simulink model "sampleModel1695_4"  (R2023a)
settings: Solver=VariableStepAuto  StartTime=0.0  StopTime=10.0  RelTol=1e-3
libraries: simulink x3, hdlsllib x3
settings Model: Creator=user1  LastModifiedBy=user1

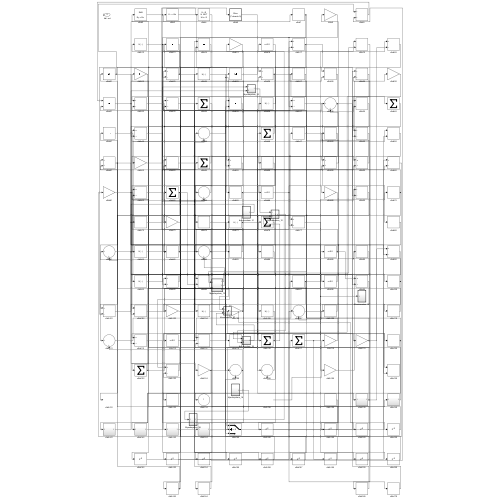
[thumbnail: Simulink's stored preview of the top-level diagram]
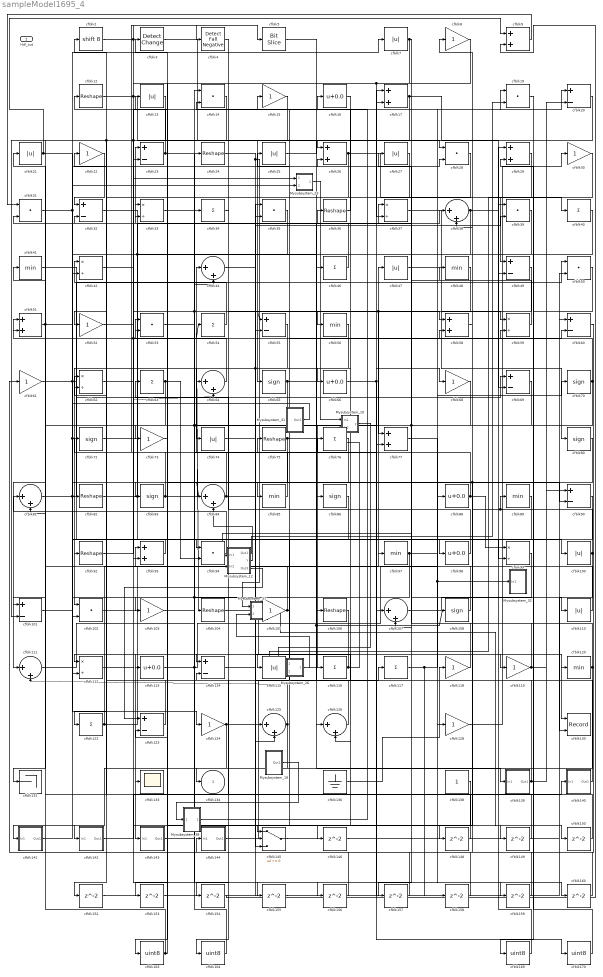
== system sampleModel1695_4 ==
  Mysubsystem_10 : Subsystem  TreatAsAtomicUnit=on  RTWFcnName=Mysubsystem_10
      settings: RTWFcnNameOpts=User specified  RTWFileNameOpts=Use function name
  Mysubsystem_12 : Subsystem  TreatAsAtomicUnit=on  RTWFcnName=Mysubsystem_12
      settings: RTWFcnNameOpts=User specified  RTWFileNameOpts=Use function name
  Mysubsystem_18 : Subsystem  TreatAsAtomicUnit=on  RTWFcnName=Mysubsystem_18
      settings: RTWFcnNameOpts=User specified  RTWFileNameOpts=Use function name
  Mysubsystem_23 : Subsystem  TreatAsAtomicUnit=on  RTWFcnName=Mysubsystem_23
      settings: RTWFcnNameOpts=User specified  RTWFileNameOpts=Use function name
  Mysubsystem_26 : Subsystem  TreatAsAtomicUnit=on  RTWFcnName=Mysubsystem_26
      settings: RTWFcnNameOpts=User specified  RTWFileNameOpts=Use function name
  Mysubsystem_31 : Subsystem  TreatAsAtomicUnit=on  RTWFcnName=Mysubsystem_31
      settings: RTWFcnNameOpts=User specified  RTWFileNameOpts=Use function name
  Mysubsystem_32 : Subsystem  TreatAsAtomicUnit=on  RTWFcnName=Mysubsystem_32
      settings: RTWFcnNameOpts=User specified  RTWFileNameOpts=Use function name
  Mysubsystem_37 : Subsystem  TreatAsAtomicUnit=on  RTWFcnName=Mysubsystem_37
      settings: RTWFcnNameOpts=User specified  RTWFileNameOpts=Use function name
  Mysubsystem_38 : Subsystem  TreatAsAtomicUnit=on  RTWFcnName=Mysubsystem_38
      settings: RTWFcnNameOpts=User specified  RTWFileNameOpts=Use function name
  cfblk{7,13,21,25,27,47,74,100,110,115} (10 alike) : Abs  OutDataTypeStr=uint8  SaturateOnIntegerOverflow=off
  cfblk{20,23,32,49,55,60,69,90,101,114,123} (11 alike) : Sum  Inputs=+-  OutDataTypeStr=uint8
  cfblk{14,19,28,31,35,39,50,53,94,102} (10 alike) : DotProduct  OutDataTypeStr=uint8
  cfblk{8,15,22,30,52,61,68,73,103,105,118..119,124,128} (14 alike) : Gain  OutDataTypeStr=uint8
  cfblk{12,24,36,75,82,92,104,106} (8 alike) : Reshape
  cfblk{38,44,64,81,84,107,111,125..126} (9 alike) : Sum  Inputs=|++  OutDataTypeStr=uint8
  cfblk{65,70,72,80,83,86,108} (7 alike) : Signum
  cfblk{33,37,42,59,62,99,112} (7 alike) : Product  Inputs=*/  OutDataTypeStr=uint8  RndMeth=Zero  SaturateOnIntegerOverflow=on
  cfblk{16,66,88,98,113} (5 alike) : Bias  Bias=0.0  SaturateOnIntegerOverflow=off
  cfblk{34,40,46,54,63,76,116..117,122} (9 alike) : Sum  Inputs=+  OutDataTypeStr=uint8
  cfblk{41,48,56,85,89,97,120} (7 alike) : MinMax  OutDataTypeStr=uint8
  cfblk130 : Record  FileSettingsInternal="{\"entries\":[{\"content\":{\"excelSettings\":{\"content\":{},\"type\":\"Streamout.ExcelSettings\"}},\"type\":\"Streamout.FileSettingStorage\",\"uuid\":\"\"}],\"packageUris\":[\"http:\\/\\/schema.mathworks.com\\/mf0\\/streamout_blocks\\/R2020a\"],\"version\":\"1.0\"}"  Layout=[1 1]  SignalsInternal="{\"entries\":[{\"content\":{\"signals\":[{\"content\":{\"blockPath\":[],\"dimensions\":[1],\"domain\":\"\",\"lineColor\":\"#a2142f\",\"plots\":[1],\"port\":1,\"signalID\":35599,\"signalName\":\"cfblk104\"},\"type\":\"RecordBlkView.Signal\",\"uuid\":\"\"},{\"content\":{\"blockPath\":[],\"dimensions\":[1],\"domain\":\"\",\"lineColor\":\"#139fff\",\"plots\":[1],\"port\":2,\"signalID\":35602,\"signalName\":\"cfblk100\"},\"type\":\"RecordBlkView.Signal\",\"uuid\":\"\"}]},\"type\":\"RecordBlkView.InputSignals\",\"uuid\":\"\"}],\"packageUris\":[\"http:\\/\\/schema.mathworks.com\\/mf0\\/streamout_blocks\\/R2020a\"],\"version\":\"1.0\"}"  VisualizationBindings="{\"xyplotplugin\":{\"info\":[{\"series\":[{\"bindingParametersList\":[{\"parameter\":\"X-Axis\",\"signalID\":35599,\"signalName\":\"cfblk104\"},{\"parameter\":\"Y-Axis\",\"signalID\":35602,\"signalName\":\"cfblk100\"}],\"seriesID\":21196}],\"subplotID\":1}]}}"  CompatibilityTag=XY  st=-1
  cfblk131 : Terminator
  cfblk133 : Scope
  cfblk136 : Ground
  cfblk138 : Constant  OutDataTypeStr=uint8  SampleTime=-1
  cfblk139 : Subsystem
      settings: LibrarySourceBlock=|
      | hdlsllib/Ports &
      | Subsystems/Subsystem
  cfblk140 : Subsystem
      settings: LibrarySourceBlock=|
      | hdlsllib/Ports &
      | Subsystems/Subsystem
  cfblk141 : Subsystem
      settings: LibrarySourceBlock=|
      | hdlsllib/Ports &
      | Subsystems/Subsystem
  cfblk142 : Subsystem
      settings: LibrarySourceBlock=|
      | hdlsllib/Ports &
      | Subsystems/Subsystem
  cfblk143 : Subsystem
      settings: LibrarySourceBlock=|
      | hdlsllib/Ports &
      | Subsystems/Subsystem
  cfblk144 : Subsystem
      settings: LibrarySourceBlock=|
      | hdlsllib/Ports &
      | Subsystems/Subsystem
  cfblk145 : Switch  OutDataTypeStr=uint8  SaturateOnIntegerOverflow=off  InputSameDT=off
  cfblk{146,148..150,152..160} (13 alike) : Delay  SampleTime=1
  cfblk{163..164,169..170} (4 alike) : DataTypeConversion  OutDataTypeStr=uint8  SaturateOnIntegerOverflow=off  RndMeth=Floor
  cfblk{9,17,26,29,51,58,77,93} (8 alike) : Sum  OutDataTypeStr=uint8
  cfblk2 : ArithShift  BitShiftNumber=8
  cfblk3 : simulink/Logic and Bit Operations/Detect Change  vinit=0  OutDataTypeStr=uint8
      settings: LibrarySourceBlock=|
      | hdlsllib/Logic and Bit
      | Operations/Detect
      | Change
  cfblk4 : hdlsllib/Logic and Bit Operations/Detect Fall Negative  vinit=0  OutDataTypeStr=uint8
  cfblk5 : hdlsllib/Logic and Bit Operations/Bit Slice  lidx=7  ridx=0
  cfblk134 : Outport  OutDataTypeStr=uint8  VectorParamsAs1DForOutWhenUnconnected=off
  Hdl_out : Outport  Port=2  OutDataTypeStr=uint8
  wires:
  cfblk119/1 -> cfblk93/1, cfblk20/2
  cfblk126/1 -> cfblk3/1
  cfblk83/1 -> cfblk5/1, cfblk17/2
  cfblk50/1 -> cfblk115/1
  cfblk85/1 -> cfblk44/1
  cfblk125/1 -> cfblk141/1(In1), cfblk111/2
  cfblk106/1 -> cfblk143/1(In1)
  cfblk102/1 -> cfblk47/1
  cfblk3/1 -> cfblk26/1
  cfblk107/1 -> cfblk110/1
  cfblk41/1 -> cfblk98/1
  cfblk81/1 -> cfblk50/1, cfblk99/2
  cfblk54/1 -> cfblk42/1
  cfblk46/1 -> cfblk23/1
  cfblk124/1 -> cfblk134/1, cfblk117/1
  cfblk139/1(Out1) -> cfblk75/1, cfblk90/1
  cfblk88/1 -> cfblk2/1, cfblk99/1
  cfblk53/1 -> cfblk34/1
  cfblk48/1 -> cfblk77/1, cfblk126/2
  cfblk145/1 -> cfblk50/2
  cfblk39/1 -> cfblk42/2
  cfblk56/1 -> cfblk102/1
  cfblk128/1 -> cfblk30/1
  cfblk138/1 -> cfblk61/1
  cfblk140/1(Out1) -> cfblk62/1
  cfblk51/1 -> cfblk111/1, cfblk83/1
  cfblk89/1 -> cfblk102/2
  cfblk8/1 -> cfblk93/2
  cfblk62/1 -> Mysubsystem_23/1(In1), cfblk54/1
  cfblk68/1 -> cfblk116/1
  cfblk117/1 -> Mysubsystem_32/1(In1), cfblk70/1, cfblk158/1
  cfblk55/1 -> cfblk104/1, cfblk145/2
  cfblk16/1 -> cfblk66/1
  cfblk58/1 -> cfblk8/1
  cfblk26/1 -> cfblk40/1, cfblk73/1
  cfblk60/1 -> cfblk144/1(In1)
  cfblk72/1 -> cfblk36/1
  cfblk30/1 -> cfblk49/1
  cfblk123/1 -> cfblk22/1
  cfblk21/1 -> cfblk9/1, cfblk124/1
  cfblk70/1 -> cfblk74/1, cfblk81/2, cfblk25/1
  cfblk37/1 -> cfblk59/1
  cfblk76/1 -> cfblk86/1
  cfblk144/1(Out1) -> cfblk46/1
  cfblk136/1 -> cfblk118/1
  cfblk86/1 -> cfblk145/1
  cfblk28/1 -> cfblk56/1
  cfblk32/1 -> cfblk106/1, cfblk126/1
  cfblk7/1 -> cfblk133/1, cfblk37/2, cfblk107/2
  cfblk23/1 -> cfblk12/1, cfblk156/1
  cfblk103/1 -> cfblk76/1
  cfblk122/1 -> Mysubsystem_12/2(In2), cfblk97/1
  cfblk110/1 -> cfblk53/1
  cfblk116/1 -> Mysubsystem_10/2(In2), cfblk112/1
  cfblk64/1 -> cfblk51/1
  cfblk66/1 -> cfblk68/1, cfblk170/1
  cfblk104/1 -> cfblk130/1
  cfblk63/1 -> cfblk82/1, cfblk94/2
  cfblk15/1 -> cfblk131/1, cfblk23/2
  cfblk120/1 -> cfblk142/1(In1), cfblk31/2
  cfblk52/1 -> cfblk26/2
  cfblk97/1 -> cfblk19/1, cfblk112/2
  cfblk12/1 -> cfblk65/1, cfblk155/1
  cfblk82/1 -> cfblk24/1, cfblk145/3
  cfblk142/1(Out1) -> cfblk140/1(In1)
  cfblk93/1 -> cfblk92/1
  cfblk25/1 -> cfblk28/1
  cfblk9/1 -> cfblk31/1
  cfblk80/1 -> cfblk84/1, cfblk148/1
  cfblk69/1 -> Mysubsystem_12/1(In1), cfblk94/1
  cfblk22/1 -> cfblk32/1
  cfblk27/1 -> cfblk52/1
  cfblk47/1 -> cfblk80/1
  cfblk40/1 -> cfblk122/1
  cfblk98/1 -> cfblk63/1
  cfblk65/1 -> cfblk101/1, cfblk139/1(In1)
  cfblk17/1 -> cfblk69/2, cfblk103/1
  cfblk94/1 -> cfblk21/1
  cfblk105/1 -> cfblk15/1, cfblk81/1
  cfblk92/1 -> cfblk20/1
  cfblk14/1 -> cfblk163/1
  cfblk59/1 -> cfblk27/1
  cfblk75/1 -> cfblk59/2, cfblk153/1
  cfblk100/1 -> cfblk89/1, cfblk48/1, cfblk130/2
  cfblk73/1 -> cfblk13/1
  cfblk5/1 -> cfblk119/1
  cfblk111/1 -> cfblk44/2
  cfblk113/1 -> cfblk88/1, cfblk58/2
  cfblk115/1 -> cfblk108/1, cfblk37/1
  cfblk2/1 -> cfblk4/1, cfblk64/2
  cfblk44/1 -> cfblk39/2
  cfblk24/1 -> Mysubsystem_37/1(In1), cfblk125/1
  cfblk74/1 -> cfblk120/1
  cfblk38/1 -> cfblk49/2, cfblk55/2
  cfblk143/1(Out1) -> cfblk38/1
  cfblk118/1 -> cfblk33/1
  cfblk13/1 -> cfblk101/2, cfblk152/1
  cfblk61/1 -> cfblk128/1, cfblk100/1
  cfblk49/1 -> cfblk114/1
  cfblk31/1 -> cfblk28/2, cfblk90/2
  cfblk33/1 -> cfblk105/1, cfblk159/1, cfblk77/2, cfblk55/1
  cfblk108/1 -> cfblk62/2
  cfblk34/1 -> cfblk64/1
  cfblk42/1 -> cfblk58/1
  cfblk36/1 -> cfblk16/1
  cfblk141/1(Out1) -> cfblk7/1
  cfblk84/1 -> cfblk72/1, cfblk60/2
  cfblk114/1 -> cfblk35/2
  cfblk35/1 -> cfblk113/1
  cfblk20/1 -> cfblk146/1
  cfblk146/1 -> cfblk39/1
  cfblk148/1 -> cfblk51/2
  cfblk149/1 -> cfblk114/2
  cfblk112/1 -> cfblk150/1
  cfblk150/1 -> cfblk32/2
  cfblk152/1 -> cfblk107/1
  cfblk153/1 -> cfblk125/2
  cfblk90/1 -> cfblk154/1
  cfblk154/1 -> cfblk9/2
  cfblk155/1 -> cfblk60/1
  cfblk156/1 -> cfblk123/2
  cfblk99/1 -> cfblk157/1
  cfblk157/1 -> cfblk17/1
  cfblk158/1 -> cfblk53/2
  cfblk159/1 -> cfblk38/2
  cfblk77/1 -> cfblk160/1
  cfblk160/1 -> cfblk35/1
  cfblk163/1 -> cfblk33/2, cfblk41/1
  cfblk4/1 -> cfblk164/1
  cfblk164/1 -> cfblk14/1
  cfblk19/1 -> cfblk169/1
  cfblk169/1 -> cfblk29/1
  cfblk170/1 -> cfblk29/2
  Mysubsystem_12/1(Out1) -> cfblk19/2
  Mysubsystem_12/2(Y) -> cfblk84/2
  Mysubsystem_12/3(Out3) -> cfblk123/1
  cfblk101/1 -> Mysubsystem_23/2(In2)
  Mysubsystem_23/1(Out1) -> Mysubsystem_10/1(In1)
  cfblk29/1 -> Mysubsystem_26/1(In1)
  Mysubsystem_10/1(y) -> Mysubsystem_26/2(In2)
  Mysubsystem_31/1(Out1) -> cfblk69/1, cfblk85/1
  Mysubsystem_26/1(Out1) -> Mysubsystem_37/2(In2)
  Mysubsystem_37/1(Out1) -> cfblk149/1
  Mysubsystem_18/1(Out1) -> Mysubsystem_38/1(In1)
  Mysubsystem_38/1(Out1) -> cfblk14/2

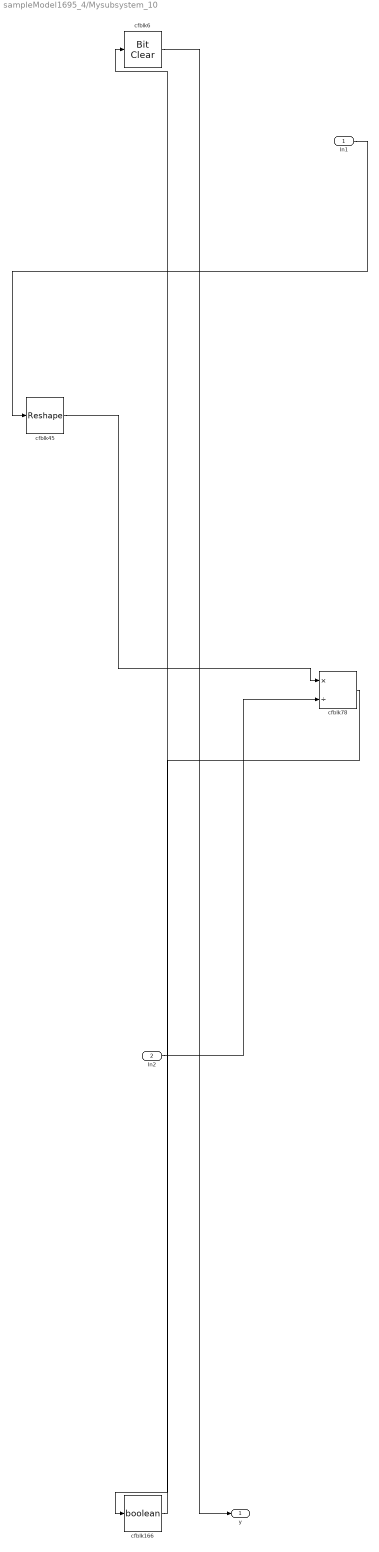
== system sampleModel1695_4/Mysubsystem_10 ==
  In1 : Inport
  In2 : Inport  Port=2
  cfblk166 : DataTypeConversion  OutDataTypeStr=boolean  SaturateOnIntegerOverflow=off  RndMeth=Floor
  cfblk45 : Reshape
  cfblk6 : simulink/Logic and Bit Operations/Bit Clear  iBit=0
      settings: LibrarySourceBlock=|
      | hdlsllib/Logic and Bit
      | Operations/Bit Clear
  cfblk78 : Product  Inputs=*/  RndMeth=Zero  SaturateOnIntegerOverflow=on
  y : Outport
  wires:
  cfblk78/1 -> cfblk166/1
  cfblk166/1 -> cfblk6/1
  In2/1 -> cfblk78/2
  cfblk45/1 -> cfblk78/1
  In1/1 -> cfblk45/1
  cfblk6/1 -> y/1

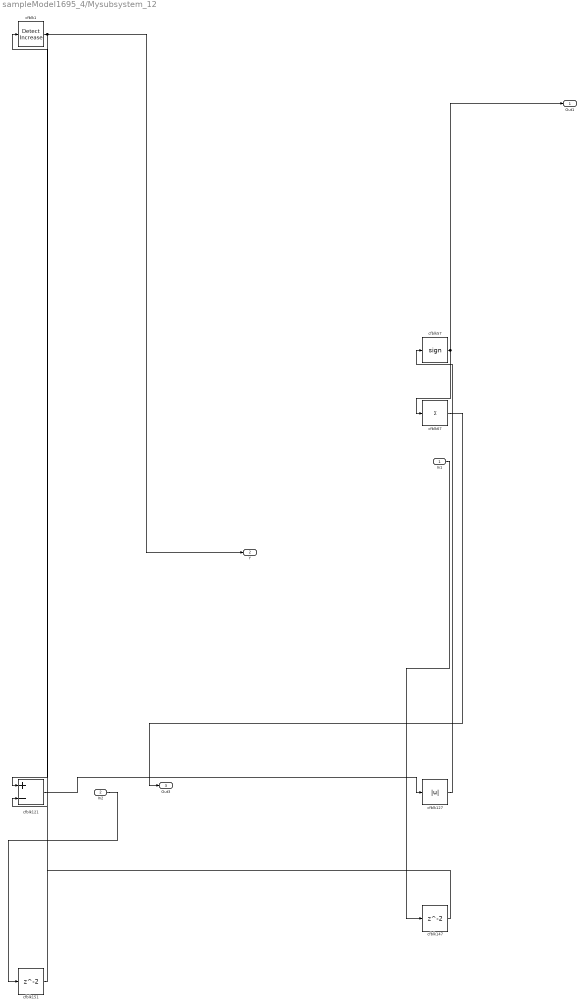
== system sampleModel1695_4/Mysubsystem_12 ==
  In1 : Inport
  In2 : Inport  Port=2
  cfblk1 : simulink/Logic and Bit Operations/Detect Increase  vinit=0.0  OutDataTypeStr=boolean
      settings: LibrarySourceBlock=|
      | hdlsllib/Logic and Bit
      | Operations/Detect
      | Increase
  cfblk121 : Sum  Inputs=+-
  cfblk127 : Abs  SaturateOnIntegerOverflow=off
  cfblk147 : Delay  SampleTime=1
  cfblk151 : Delay  SampleTime=1
  cfblk57 : Signum
  cfblk67 : Sum  Inputs=+
  Out1 : Outport
  Y : Outport  Port=2
  Out3 : Outport  Port=3
  wires:
  cfblk1/1 -> Y/1, cfblk121/1
  cfblk151/1 -> cfblk121/2
  cfblk57/1 -> Out1/1, cfblk67/1
  cfblk127/1 -> cfblk57/1
  In2/1 -> cfblk151/1
  cfblk147/1 -> cfblk1/1
  cfblk121/1 -> cfblk127/1
  In1/1 -> cfblk147/1
  cfblk67/1 -> Out3/1

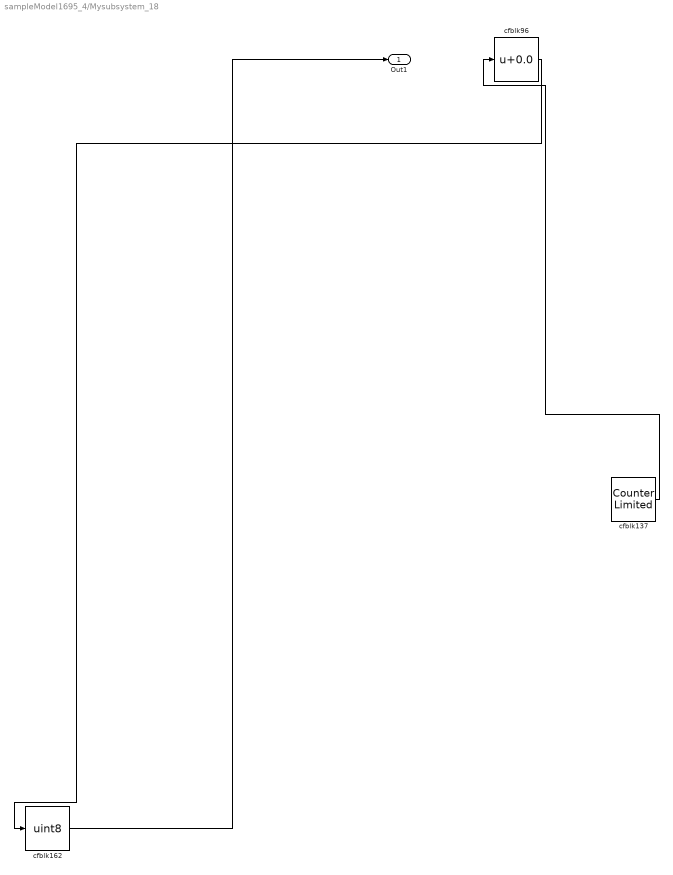
== system sampleModel1695_4/Mysubsystem_18 ==
  cfblk137 : hdlsllib/Sources/Counter Limited  uplimit=7  tsamp=-1
  cfblk162 : DataTypeConversion  OutDataTypeStr=uint8  SaturateOnIntegerOverflow=off  RndMeth=Floor
  cfblk96 : Bias  Bias=0.0  SaturateOnIntegerOverflow=off
  Out1 : Outport
  wires:
  cfblk96/1 -> cfblk162/1
  cfblk137/1 -> cfblk96/1
  cfblk162/1 -> Out1/1

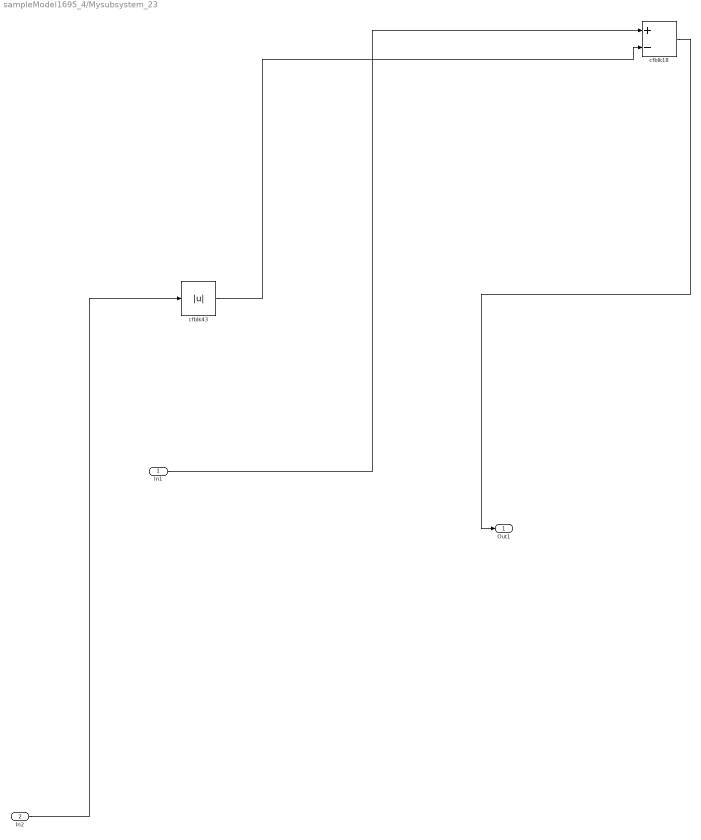
== system sampleModel1695_4/Mysubsystem_23 ==
  In1 : Inport
  In2 : Inport  Port=2
  cfblk18 : Sum  Inputs=+-
  cfblk43 : Abs  SaturateOnIntegerOverflow=off
  Out1 : Outport
  wires:
  cfblk43/1 -> cfblk18/2
  cfblk18/1 -> Out1/1
  In1/1 -> cfblk18/1
  In2/1 -> cfblk43/1

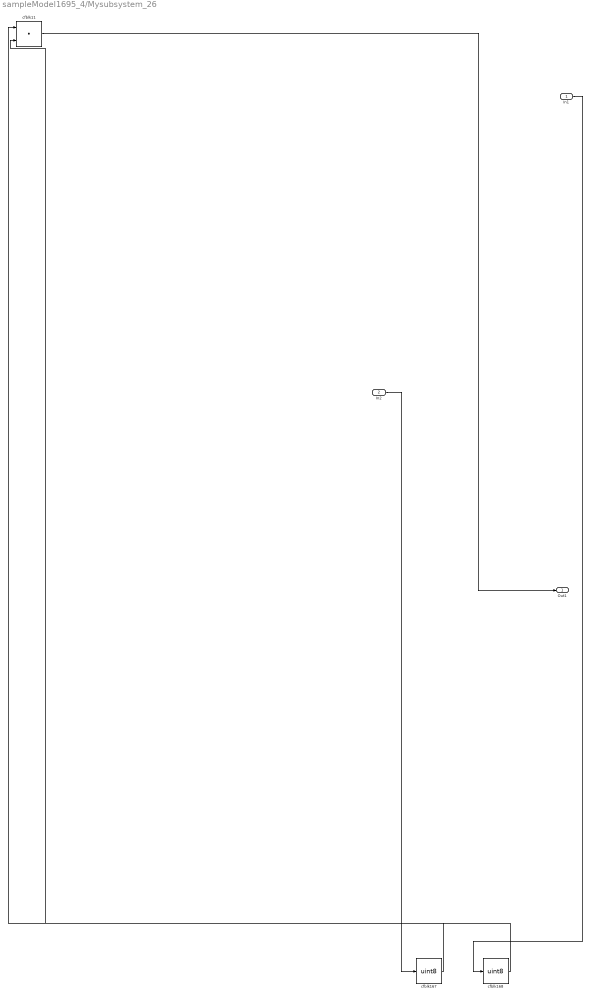
== system sampleModel1695_4/Mysubsystem_26 ==
  In1 : Inport
  In2 : Inport  Port=2
  cfblk11 : DotProduct  OutDataTypeStr=Inherit: Inherit via internal rule
  cfblk167 : DataTypeConversion  OutDataTypeStr=uint8  SaturateOnIntegerOverflow=off  RndMeth=Floor
  cfblk168 : DataTypeConversion  OutDataTypeStr=uint8  SaturateOnIntegerOverflow=off  RndMeth=Floor
  Out1 : Outport
  wires:
  In2/1 -> cfblk167/1
  cfblk167/1 -> cfblk11/2
  cfblk168/1 -> cfblk11/1
  In1/1 -> cfblk168/1
  cfblk11/1 -> Out1/1

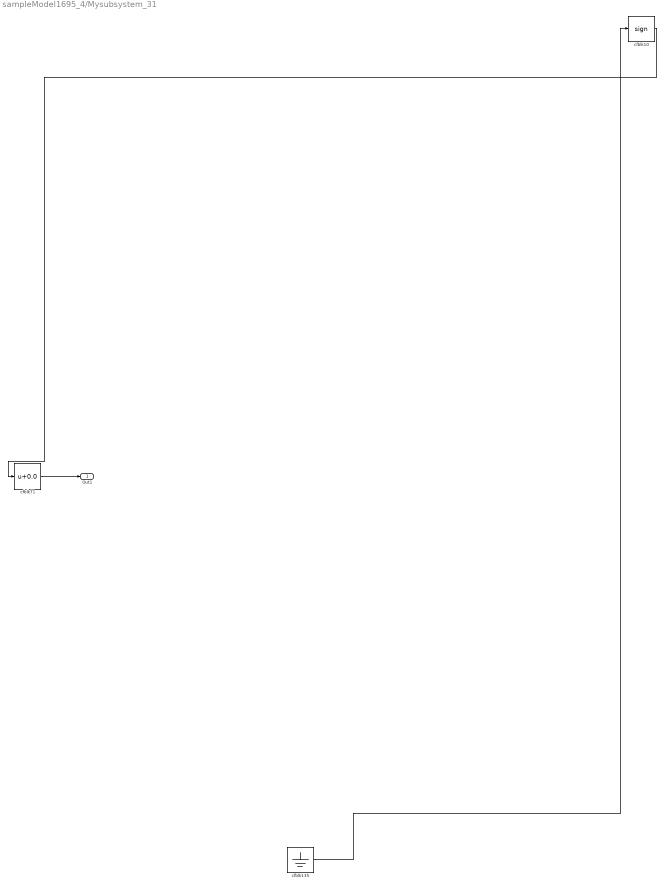
== system sampleModel1695_4/Mysubsystem_31 ==
  cfblk10 : Signum
  cfblk135 : Ground
  cfblk71 : Bias  Bias=0.0  SaturateOnIntegerOverflow=off
  Out1 : Outport
  wires:
  cfblk10/1 -> cfblk71/1
  cfblk135/1 -> cfblk10/1
  cfblk71/1 -> Out1/1

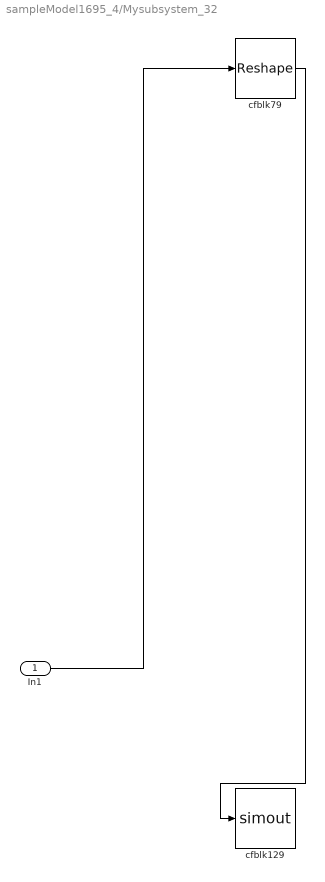
== system sampleModel1695_4/Mysubsystem_32 ==
  In1 : Inport
  cfblk129 : ToWorkspace  VariableName=simout  SaveFormat=Timeseries  SampleTime=-1
  cfblk79 : Reshape
  wires:
  cfblk79/1 -> cfblk129/1
  In1/1 -> cfblk79/1

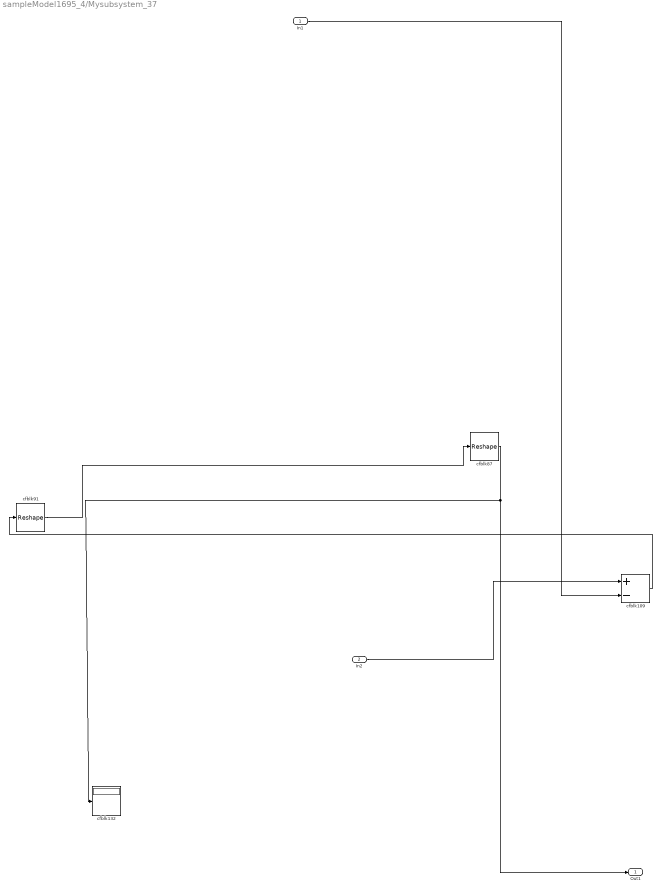
== system sampleModel1695_4/Mysubsystem_37 ==
  In1 : Inport
  In2 : Inport  Port=2
  cfblk109 : Sum  Inputs=+-
  cfblk132 : Display
  cfblk87 : Reshape
  cfblk91 : Reshape
  Out1 : Outport
  wires:
  cfblk109/1 -> cfblk91/1
  cfblk87/1 -> Out1/1, cfblk132/1
  In2/1 -> cfblk109/1
  cfblk91/1 -> cfblk87/1
  In1/1 -> cfblk109/2

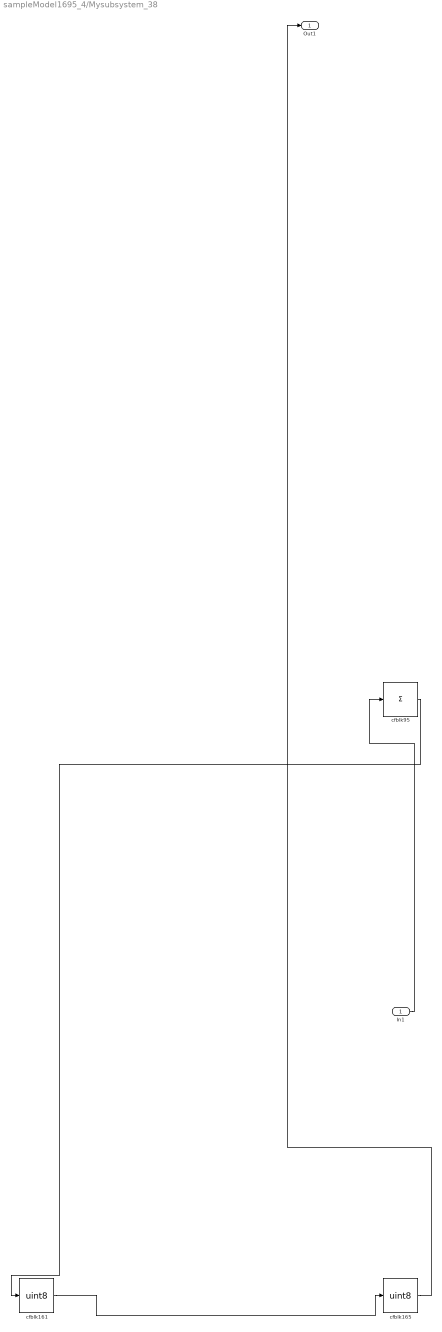
== system sampleModel1695_4/Mysubsystem_38 ==
  In1 : Inport
  cfblk161 : DataTypeConversion  OutDataTypeStr=uint8  SaturateOnIntegerOverflow=off  RndMeth=Floor
  cfblk165 : DataTypeConversion  OutDataTypeStr=uint8  SaturateOnIntegerOverflow=off  RndMeth=Floor
  cfblk95 : Sum  Inputs=+
  Out1 : Outport
  wires:
  cfblk161/1 -> cfblk165/1
  cfblk165/1 -> Out1/1
  cfblk95/1 -> cfblk161/1
  In1/1 -> cfblk95/1

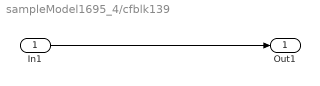
== system sampleModel1695_4/cfblk139 ==
  In1 : Inport
  Out1 : Outport
  wires:
  In1/1 -> Out1/1

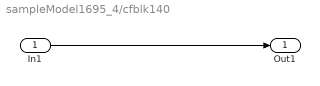
== system sampleModel1695_4/cfblk140 ==
  In1 : Inport
  Out1 : Outport
  wires:
  In1/1 -> Out1/1

== system sampleModel1695_4/cfblk141 ==
  In1 : Inport
  Out1 : Outport
  wires:
  In1/1 -> Out1/1

== system sampleModel1695_4/cfblk142 ==
  In1 : Inport
  Out1 : Outport
  wires:
  In1/1 -> Out1/1

== system sampleModel1695_4/cfblk143 ==
  In1 : Inport
  Out1 : Outport
  wires:
  In1/1 -> Out1/1

== system sampleModel1695_4/cfblk144 ==
  In1 : Inport
  Out1 : Outport
  wires:
  In1/1 -> Out1/1
